simulink library "atmospheric_library"  (R2017a)
settings: Solver=VariableStepAuto  StartTime=0.0  StopTime=10.0  RelTol=1e-3
libraries: simulink x2
settings Model: Creator=marriott  LastModifiedBy=marriott
settings OptimizationCC: LifeSpan=inf
settings DebuggingCC: SFExecutionAtInitializationDiag=none

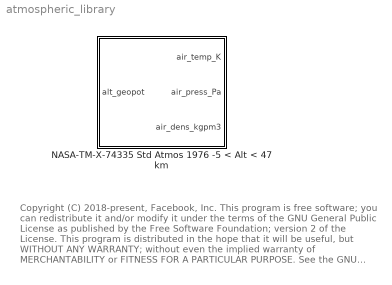
== system atmospheric_library ==
  note: Copyright (C) 2018-present, Facebook, Inc.
      |
      | This program is free software; you can redistribute it and/or modify
      | it under the terms of the GNU General Public License as published by
      | the Free Software Foundation; version 2 of the License.
      |
      | This program is distributed in the hope that it will be useful,
      | but WITHOUT ANY WARRANTY; without even the implied warranty of
      | MERCHANTABILITY or FITNESS FOR A PARTICULAR PURPOSE. See the
      | GNU General Public License for more details.
      |
      | You should have received a copy of the GNU General Public License along
      | with this program; if not, write to the Free Software Foundation, Inc.,
      | 51 Franklin Street, Fifth Floor, Boston, MA 02110-1301 USA.
  NASA-TM-X-74335 Std Atmos 1976 -5 < Alt < 47 km : Subsystem

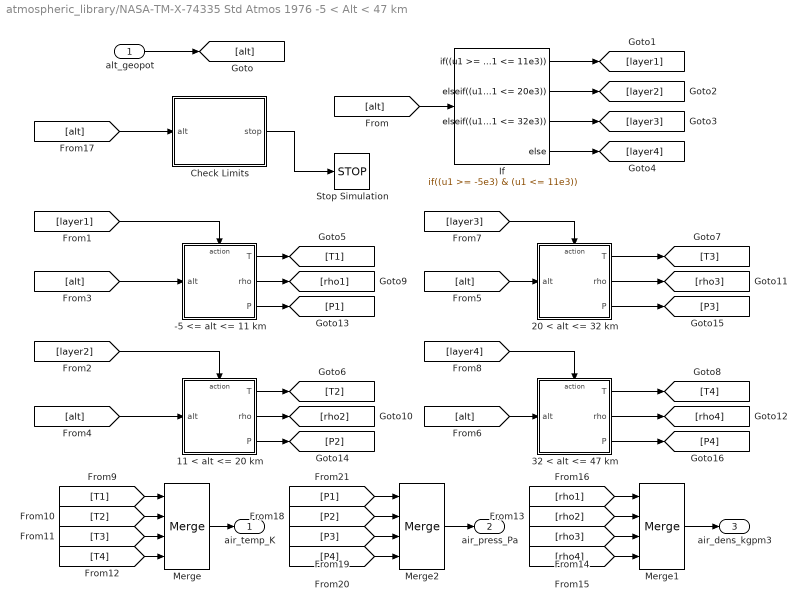
== system atmospheric_library/NASA-TM-X-74335 Std Atmos 1976 -5 < Alt < 47 km ==
  alt_geopot : Inport
  -5 <= alt <= 11 km : Subsystem  TreatAsAtomicUnit=on
  11 < alt <= 20 km : Subsystem  TreatAsAtomicUnit=on
  20 < alt <= 32 km : Subsystem  TreatAsAtomicUnit=on
  32 < alt <= 47 km : Subsystem  TreatAsAtomicUnit=on
  Check Limits : Subsystem
  If : If  IfExpression=(u1 >= -5e3) & (u1 <= 11e3)  ElseIfExpressions=(u1 > 11e3) & (u1 <= 20e3),(u1 > 20e3) & (u1 <= 32e3)
  Merge : Merge  Inputs=4
  Merge1 : Merge  Inputs=4
  Merge2 : Merge  Inputs=4
  Stop Simulation : Stop
  air_temp_K : Outport
  air_press_Pa : Outport  Port=2
  air_dens_kgpm3 : Outport  Port=3
  wires:
  Merge1/1 -> air_dens_kgpm3/1
  [T2] -> Merge/2
  [T3] -> Merge/3
  [T4] -> Merge/4
  [rho3] -> Merge1/3
  [rho4] -> Merge1/4
  [rho1] -> Merge1/1
  [rho2] -> Merge1/2
  Merge/1 -> air_temp_K/1
  [alt] -> -5 <= alt <= 11 km/1(alt)
  If/1 -> [layer1]
  [alt] -> If/1
  alt_geopot/1 -> [alt]
  If/2 -> [layer2]
  If/3 -> [layer3]
  If/4 -> [layer4]
  [layer1] -> -5 <= alt <= 11 km/Action
  [T1] -> Merge/1
  [alt] -> Check Limits/1(alt)
  Check Limits/1(stop) -> Stop Simulation/1
  [layer2] -> 11 < alt <= 20 km/Action
  [alt] -> 11 < alt <= 20 km/1(alt)
  [layer3] -> 20 < alt <= 32 km/Action
  [layer4] -> 32 < alt <= 47 km/Action
  [alt] -> 20 < alt <= 32 km/1(alt)
  [alt] -> 32 < alt <= 47 km/1(alt)
  -5 <= alt <= 11 km/1(T) -> [T1]
  -5 <= alt <= 11 km/2(rho) -> [rho1]
  -5 <= alt <= 11 km/3(P) -> [P1]
  11 < alt <= 20 km/1(T) -> [T2]
  11 < alt <= 20 km/2(rho) -> [rho2]
  11 < alt <= 20 km/3(P) -> [P2]
  20 < alt <= 32 km/1(T) -> [T3]
  20 < alt <= 32 km/2(rho) -> [rho3]
  20 < alt <= 32 km/3(P) -> [P3]
  32 < alt <= 47 km/1(T) -> [T4]
  32 < alt <= 47 km/2(rho) -> [rho4]
  32 < alt <= 47 km/3(P) -> [P4]
  Merge2/1 -> air_press_Pa/1
  [P1] -> Merge2/1
  [P2] -> Merge2/2
  [P3] -> Merge2/3
  [P4] -> Merge2/4

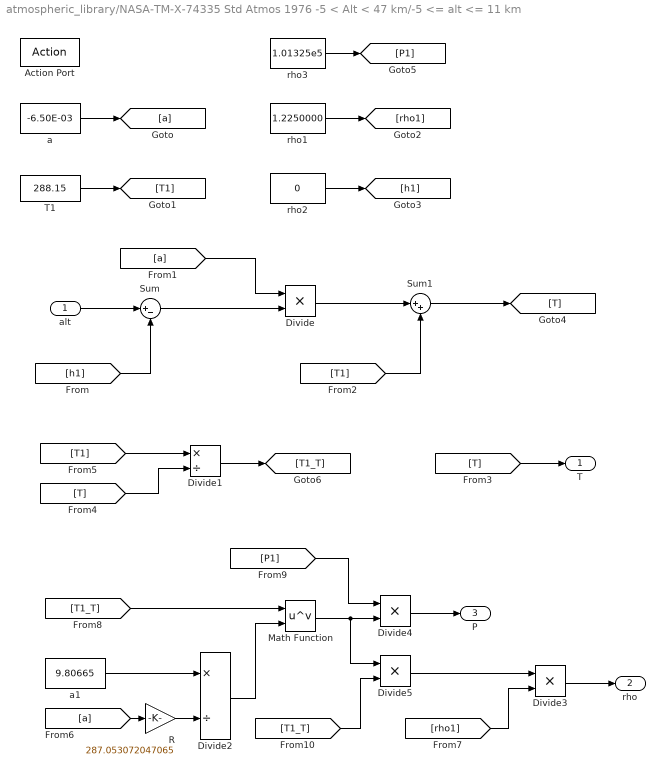
== system atmospheric_library/NASA-TM-X-74335 Std Atmos 1976 -5 < Alt < 47 km/-5 <= alt <= 11 km ==
  alt : Inport
  Action Port : ActionPort
  Divide{,3..5} (4 alike) : Product  Inputs=**
  Divide1 : Product  Inputs=*/
  Divide2 : Product  Inputs=*/
  Math Function : Math  Operator=pow  SaturateOnIntegerOverflow=on
  R : Gain  Gain=287.053072047065
  Sum : Sum  Inputs=|+-
  Sum1 : Sum  Inputs=|++
  T1 : Constant  Value=288.15
  a : Constant  Value=-6.50E-03
  a1 : Constant  Value=9.80665
  rho1 : Constant  Value=1.2250000
  rho2 : Constant  Value=0
  rho3 : Constant  Value=1.01325e5
  T : Outport
  rho : Outport  Port=2
  P : Outport  Port=3
  wires:
  a/1 -> [a]
  T1/1 -> [T1]
  rho1/1 -> [rho1]
  rho2/1 -> [h1]
  alt/1 -> Sum/1
  [h1] -> Sum/2
  Divide/1 -> Sum1/1
  [T1] -> Sum1/2
  Sum1/1 -> [T]
  [T] -> T/1
  Sum/1 -> Divide/2
  [a] -> Divide/1
  [a] -> R/1
  a1/1 -> Divide2/1
  R/1 -> Divide2/2
  Divide3/1 -> rho/1
  rho3/1 -> [P1]
  [T1] -> Divide1/1
  [T] -> Divide1/2
  Divide1/1 -> [T1_T]
  [T1_T] -> Math Function/1
  Divide2/1 -> Math Function/2
  Math Function/1 -> Divide5/1, Divide4/2
  [P1] -> Divide4/1
  Divide4/1 -> P/1
  [T1_T] -> Divide5/2
  Divide5/1 -> Divide3/1
  [rho1] -> Divide3/2

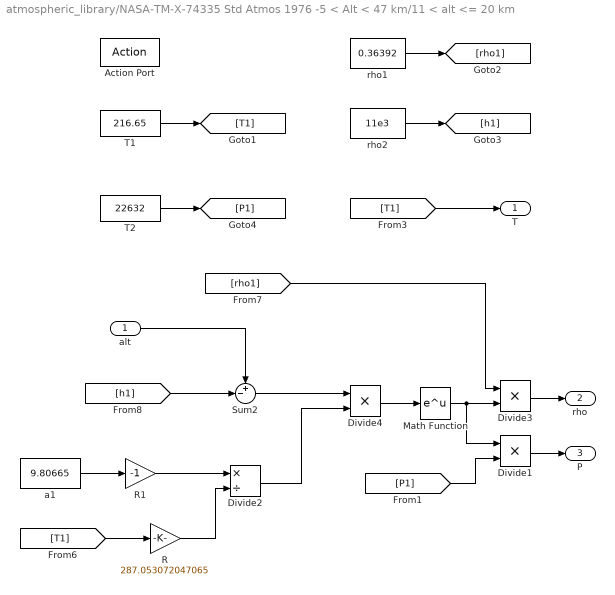
== system atmospheric_library/NASA-TM-X-74335 Std Atmos 1976 -5 < Alt < 47 km/11 < alt <= 20 km ==
  alt : Inport
  Action Port : ActionPort
  Divide1 : Product  Inputs=**
  Divide2 : Product  Inputs=*/
  Divide3 : Product  Inputs=**
  Divide4 : Product  Inputs=**
  Math Function : Math  SaturateOnIntegerOverflow=on
  R : Gain  Gain=287.053072047065
  R1 : Gain  Gain=-1
  Sum2 : Sum  Inputs=+-|
  T1 : Constant  Value=216.65
  T2 : Constant  Value=22632
  a1 : Constant  Value=9.80665
  rho1 : Constant  Value=0.36392
  rho2 : Constant  Value=11e3
  T : Outport
  rho : Outport  Port=2
  P : Outport  Port=3
  wires:
  T1/1 -> [T1]
  rho1/1 -> [rho1]
  rho2/1 -> [h1]
  [T1] -> T/1
  [T1] -> R/1
  a1/1 -> R1/1
  R/1 -> Divide2/2
  Math Function/1 -> Divide1/1, Divide3/2
  [rho1] -> Divide3/1
  Divide3/1 -> rho/1
  alt/1 -> Sum2/1
  [h1] -> Sum2/2
  Sum2/1 -> Divide4/1
  Divide2/1 -> Divide4/2
  R1/1 -> Divide2/1
  Divide4/1 -> Math Function/1
  Divide1/1 -> P/1
  T2/1 -> [P1]
  [P1] -> Divide1/2

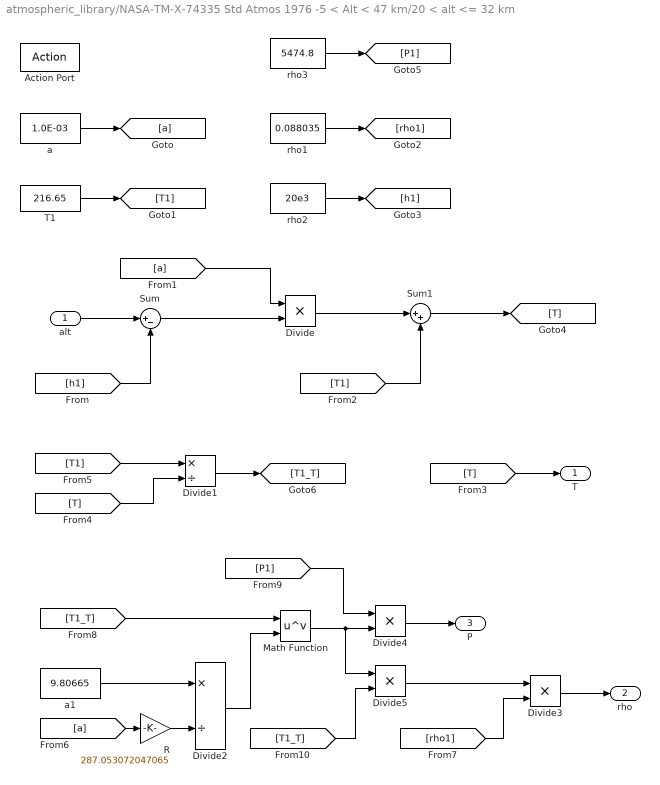
== system atmospheric_library/NASA-TM-X-74335 Std Atmos 1976 -5 < Alt < 47 km/20 < alt <= 32 km ==
  alt : Inport
  Action Port : ActionPort
  Divide{,3..5} (4 alike) : Product  Inputs=**
  Divide1 : Product  Inputs=*/
  Divide2 : Product  Inputs=*/
  Math Function : Math  Operator=pow  SaturateOnIntegerOverflow=on
  R : Gain  Gain=287.053072047065
  Sum : Sum  Inputs=|+-
  Sum1 : Sum  Inputs=|++
  T1 : Constant  Value=216.65
  a : Constant  Value=1.0E-03
  a1 : Constant  Value=9.80665
  rho1 : Constant  Value=0.088035
  rho2 : Constant  Value=20e3
  rho3 : Constant  Value=5474.8
  T : Outport
  rho : Outport  Port=2
  P : Outport  Port=3
  wires:
  a/1 -> [a]
  T1/1 -> [T1]
  rho1/1 -> [rho1]
  rho2/1 -> [h1]
  alt/1 -> Sum/1
  [h1] -> Sum/2
  Divide/1 -> Sum1/1
  [T1] -> Sum1/2
  Sum1/1 -> [T]
  Sum/1 -> Divide/2
  [a] -> Divide/1
  rho3/1 -> [P1]
  [T] -> T/1
  [a] -> R/1
  a1/1 -> Divide2/1
  R/1 -> Divide2/2
  Divide3/1 -> rho/1
  [T1] -> Divide1/1
  [T] -> Divide1/2
  Divide1/1 -> [T1_T]
  [T1_T] -> Math Function/1
  Divide2/1 -> Math Function/2
  Math Function/1 -> Divide5/1, Divide4/2
  [P1] -> Divide4/1
  Divide4/1 -> P/1
  [T1_T] -> Divide5/2
  Divide5/1 -> Divide3/1
  [rho1] -> Divide3/2

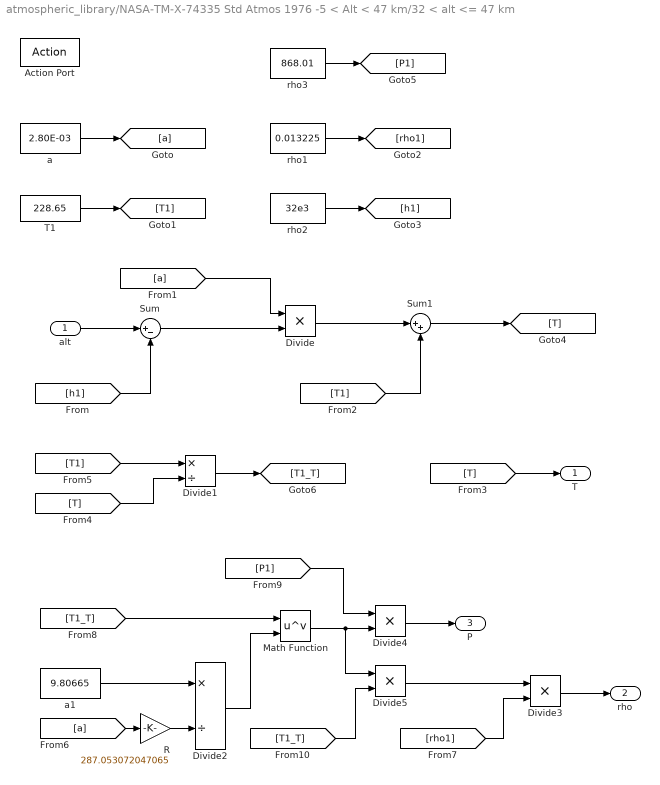
== system atmospheric_library/NASA-TM-X-74335 Std Atmos 1976 -5 < Alt < 47 km/32 < alt <= 47 km ==
  alt : Inport
  Action Port : ActionPort
  Divide{,3..5} (4 alike) : Product  Inputs=**
  Divide1 : Product  Inputs=*/
  Divide2 : Product  Inputs=*/
  Math Function : Math  Operator=pow  SaturateOnIntegerOverflow=on
  R : Gain  Gain=287.053072047065
  Sum : Sum  Inputs=|+-
  Sum1 : Sum  Inputs=|++
  T1 : Constant  Value=228.65
  a : Constant  Value=2.80E-03
  a1 : Constant  Value=9.80665
  rho1 : Constant  Value=0.013225
  rho2 : Constant  Value=32e3
  rho3 : Constant  Value=868.01
  T : Outport
  rho : Outport  Port=2
  P : Outport  Port=3
  wires:
  a/1 -> [a]
  T1/1 -> [T1]
  rho1/1 -> [rho1]
  rho2/1 -> [h1]
  alt/1 -> Sum/1
  [h1] -> Sum/2
  Divide/1 -> Sum1/1
  [T1] -> Sum1/2
  Sum1/1 -> [T]
  Sum/1 -> Divide/2
  [a] -> Divide/1
  rho3/1 -> [P1]
  [T] -> T/1
  [a] -> R/1
  a1/1 -> Divide2/1
  R/1 -> Divide2/2
  Divide3/1 -> rho/1
  [T1] -> Divide1/1
  [T] -> Divide1/2
  Divide1/1 -> [T1_T]
  [T1_T] -> Math Function/1
  Divide2/1 -> Math Function/2
  Math Function/1 -> Divide5/1, Divide4/2
  [P1] -> Divide4/1
  Divide4/1 -> P/1
  [T1_T] -> Divide5/2
  Divide5/1 -> Divide3/1
  [rho1] -> Divide3/2

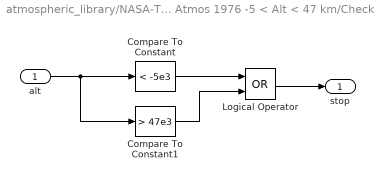
== system atmospheric_library/NASA-TM-X-74335 Std Atmos 1976 -5 < Alt < 47 km/Check Limits ==
  alt : Inport
  Compare To Constant : simulink/Logic and Bit Operations/Compare To Constant  relop=<  const=-5e3  OutDataTypeStr=boolean
  Compare To Constant1 : simulink/Logic and Bit Operations/Compare To Constant  relop=>  const=47e3  OutDataTypeStr=boolean
  Logical Operator : Logic  Operator=OR  AllPortsSameDT=off  OutDataTypeStr=boolean
  stop : Outport
  wires:
  Compare To Constant1/1 -> Logical Operator/2
  Logical Operator/1 -> stop/1
  Compare To Constant/1 -> Logical Operator/1
  alt/1 -> Compare To Constant1/1, Compare To Constant/1
